simulink model "HoldLogic"  (R2024b)
settings: Solver=FixedStepAuto  StartTime=0.0  StopTime=inf  FixedStep=0.004  RelTol=1e-3
settings Model: Creator=StefanoLucaParravici  LastModifiedBy=StefanoLucaParravici

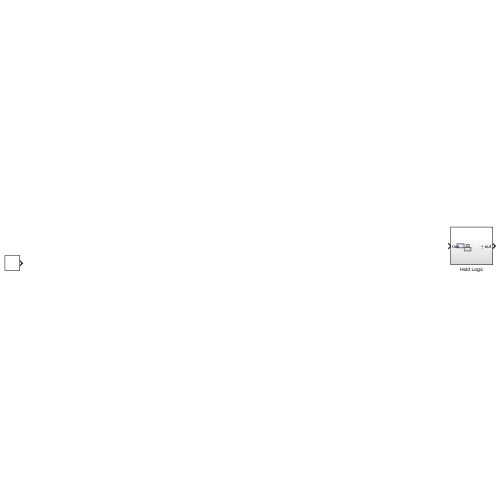
[thumbnail: Simulink's stored preview of the top-level diagram]
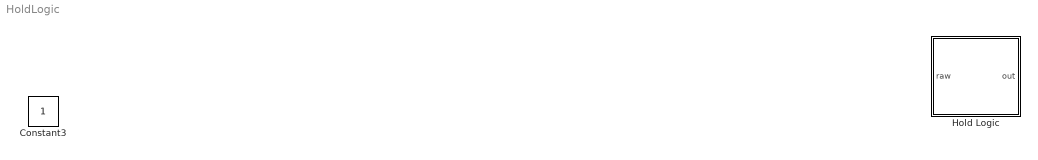
== system HoldLogic ==
  Constant3 : Constant
  Hold Logic : Subsystem

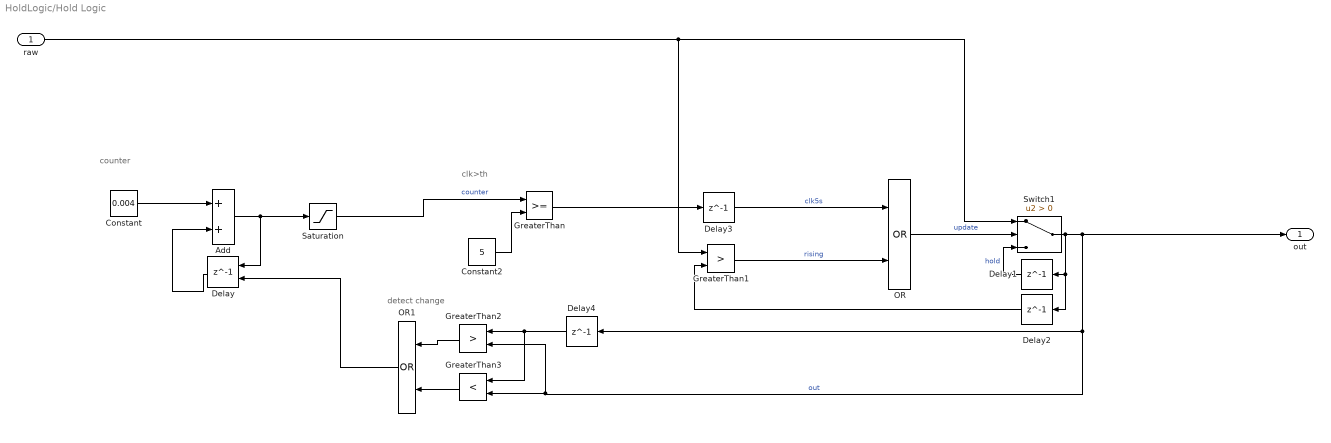
== system HoldLogic/Hold Logic ==
  note: detect change
  note: clk>th
  note: counter
  raw : Inport
  Add : Sum
  Constant : Constant  Value=0.004  OutDataTypeStr=single
  Constant2 : Constant  Value=5
  Delay : Delay  DelayLength=1  ExternalReset=Rising
      settings: InputPortMap=u0,r5
  Delay{1..4} (4 alike) : Delay  DelayLength=1
  GreaterThan : RelationalOperator  OutDataTypeStr=boolean  RndMeth=Simplest  InputSameDT=off
  GreaterThan1 : RelationalOperator  Operator=>  OutDataTypeStr=boolean  RndMeth=Simplest  InputSameDT=off
  GreaterThan2 : RelationalOperator  Operator=>  OutDataTypeStr=boolean  RndMeth=Simplest  InputSameDT=off
  GreaterThan3 : RelationalOperator  Operator=<  OutDataTypeStr=boolean  RndMeth=Simplest  InputSameDT=off
  OR : Logic  Operator=OR  AllPortsSameDT=off  OutDataTypeStr=boolean
  OR1 : Logic  Operator=OR  AllPortsSameDT=off  OutDataTypeStr=boolean
  Saturation : Saturate  UpperLimit=10  LowerLimit=0
  Switch1 : Switch  Criteria=u2 > Threshold  SaturateOnIntegerOverflow=off  InputSameDT=off
  out : Outport
  wires:
  GreaterThan/1 -> Delay3/1
  Delay4/1 -> GreaterThan3/1, GreaterThan2/1
  Constant2/1 -> GreaterThan/2
  GreaterThan1/1 -> OR/2  "rising"
  Constant/1 -> Add/1
  Switch1/1 -> Delay2/1, Delay1/1, GreaterThan2/2, GreaterThan3/2, Delay4/1, out/1  "out"
  GreaterThan3/1 -> OR1/2
  OR1/1 -> Delay/2
  raw/1 -> GreaterThan1/1, Switch1/1
  Saturation/1 -> GreaterThan/1  "counter"
  Delay/1 -> Add/2
  Add/1 -> Saturation/1, Delay/1
  GreaterThan2/1 -> OR1/1
  Delay2/1 -> GreaterThan1/2
  OR/1 -> Switch1/2  "update"
  Delay1/1 -> Switch1/3  "hold"
  Delay3/1 -> OR/1  "clk5s"
